simulink library "CTADP_lib"  (Simulink 7.5)
settings: Solver=ode45  StartTime=0.0  StopTime=10.0  RelTol=1e-3
libraries: simulink x2
settings Model: Creator=Yuri  LastModifiedBy=Yuri

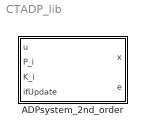
== system CTADP_lib ==
  ADPsystem_2nd_order : Subsystem  mask{K=[0,0], Q=eye(2), R=1, dT=0.1}
      mask prompts: K "Control gain K"; Q "Weight Matrix Q"; R "Weight Matrix R"; dT "Learning Interval dT"

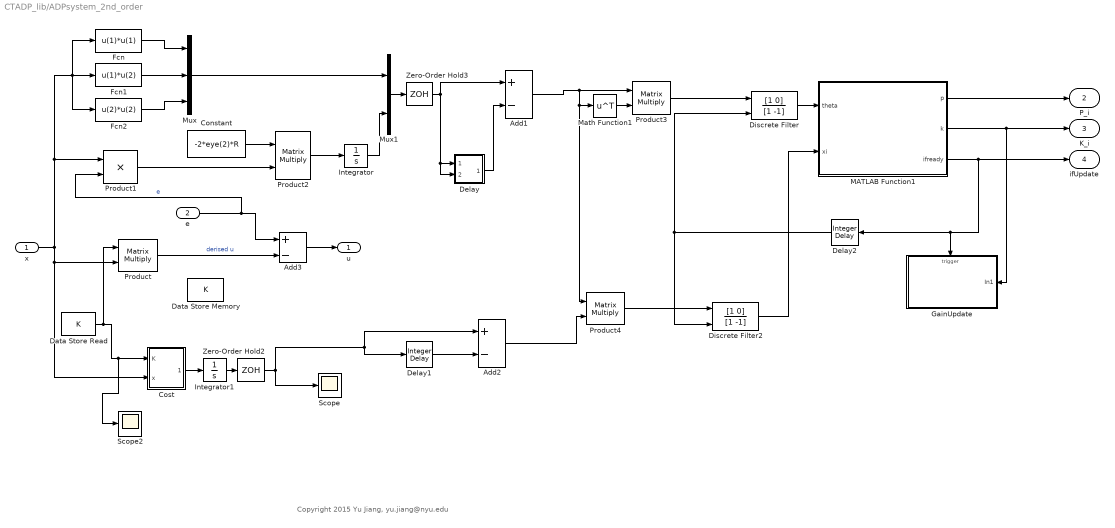
== system CTADP_lib/ADPsystem_2nd_order ==
  note: Copyright 2015 Yu Jiang, yu.jiang@nyu.edu
  x : Inport
  e : Inport  Port=2
  Add1 : Sum  Inputs=+-
  Add2 : Sum  Inputs=+-
  Add3 : Sum  Inputs=+-
  Constant : Constant  Value=-2*eye(2)*R  VectorParams1D=off
  Cost : Subsystem
  Data Store Memory : DataStoreMemory  Priority=1  DataStoreName=K  InitialValue=K  VectorParams1D=off
  Data Store Read : DataStoreRead  DataStoreName=K  SampleTime=0
  Delay : Subsystem  Description=Replaced Block
      mask Type: Replaced Block
      mask Description: SaveAs has replaced this block with an empty subsystem because the block represents a new type or uses a new functionality.
      mask Display: fprintf('Replaced: %s\n','Delay')
  Delay1 : simulink/Discrete/Integer Delay  NumDelays=1  vinit=0  samptime=dT
  Delay2 : simulink/Discrete/Integer Delay  NumDelays=1  vinit=0  samptime=dT
  Discrete Filter : DiscreteFilter  Numerator=[1 0]  Denominator=[1 -1]  SampleTime=dT  NumAccumDataTypeStr=Inherit: Same as product output  OutDataTypeStr=Inherit: Same as input
  Discrete Filter2 : DiscreteFilter  Numerator=[1 0]  Denominator=[1 -1]  SampleTime=dT  NumAccumDataTypeStr=Inherit: Same as product output  OutDataTypeStr=Inherit: Same as input
  Fcn : Fcn  Expr=u(1)*u(1)
  Fcn1 : Fcn  Expr=u(1)*u(2)
  Fcn2 : Fcn  Expr=u(2)*u(2)
  GainUpdate : Subsystem
  Integrator : Integrator
  Integrator1 : Integrator
  MATLAB Function1 : Stateflow chart  TreatAsAtomicUnit=on
      settings: PermitHierarchicalResolution=ParametersOnly
  Math Function1 : Math  Operator=transpose  SaturateOnIntegerOverflow=on
  Mux : Mux  Inputs=3
  Mux1 : Mux  Inputs=2
  Product{,2..4} (4 alike) : Product  Multiplication=Matrix(*)
  Product1 : Product
  Scope : Scope
  Scope2 : Scope
      settings: SaveName=ScopeData4
  Zero-Order Hold2 : ZeroOrderHold  SampleTime=dT
  Zero-Order Hold3 : ZeroOrderHold  SampleTime=dT
  u : Outport
  P_i : Outport  Port=2
  K_i : Outport  Port=3
  ifUpdate : Outport  Port=4
  wires:
  x/1 -> Cost/2(x), Product/2, Fcn/1, Fcn2/1, Fcn1/1, Product1/1
  Product/1 -> Add3/2  "derised u"
  Data Store Read/1 -> Scope2/1, Cost/1(K), Product/1
  Fcn1/1 -> Mux/2
  Fcn/1 -> Mux/1
  Fcn2/1 -> Mux/3
  Product1/1 -> Product2/2
  Constant/1 -> Product2/1
  Product2/1 -> Integrator/1
  Integrator/1 -> Mux1/2
  Zero-Order Hold3/1 -> Delay/2(In2), Delay/1(In1), Add1/1
  Mux/1 -> Mux1/1
  Delay/1(Out1) -> Add1/2
  Cost/1(r(x,uk)) -> Integrator1/1
  Integrator1/1 -> Zero-Order Hold2/1
  Delay1/1 -> Add2/2
  Add3/1 -> u/1
  e/1 -> Product1/2, Add3/1  "e"
  Math Function1/1 -> Product3/2
  Product3/1 -> Discrete Filter/1
  Add2/1 -> Product4/2
  Product4/1 -> Discrete Filter2/1
  Discrete Filter/1 -> MATLAB Function1/1(theta)
  Discrete Filter2/1 -> MATLAB Function1/2(xi)
  Mux1/1 -> Zero-Order Hold3/1
  Zero-Order Hold2/1 -> Scope/1, Delay1/1, Add2/1
  MATLAB Function1/3(ifready) -> ifUpdate/1, Delay2/1, GainUpdate/Trigger
  MATLAB Function1/1(p) -> P_i/1
  MATLAB Function1/2(k) -> GainUpdate/1(In1), K_i/1
  Delay2/1 -> Discrete Filter/2, Discrete Filter2/2
  Add1/1 -> Product4/1, Math Function1/1, Product3/1

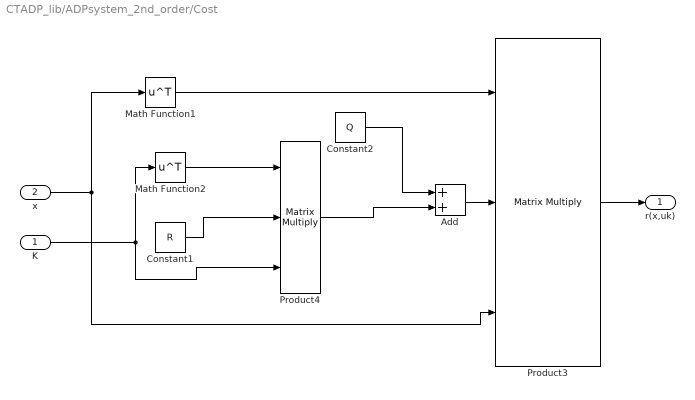
== system CTADP_lib/ADPsystem_2nd_order/Cost ==
  K : Inport
  x : Inport  Port=2
  Add : Sum
  Constant1 : Constant  Value=R
  Constant2 : Constant  Value=Q
  Math Function1 : Math  Operator=transpose  SaturateOnIntegerOverflow=on
  Math Function2 : Math  Operator=transpose  SaturateOnIntegerOverflow=on
  Product3 : Product  Inputs=3  Multiplication=Matrix(*)
  Product4 : Product  Inputs=3  Multiplication=Matrix(*)
  r(x,uk) : Outport
  wires:
  Add/1 -> Product3/2
  x/1 -> Math Function1/1, Product3/3
  Product4/1 -> Add/2
  Math Function1/1 -> Product3/1
  Product3/1 -> r(x,uk)/1
  Constant2/1 -> Add/1
  K/1 -> Math Function2/1, Product4/3
  Constant1/1 -> Product4/2
  Math Function2/1 -> Product4/1

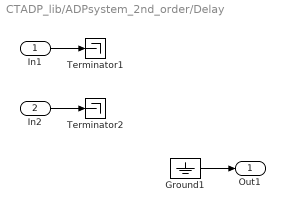
== system CTADP_lib/ADPsystem_2nd_order/Delay ==
  In1 : Inport
  In2 : Inport  Port=2
  Ground1 : Ground
  Terminator1 : Terminator
  Terminator2 : Terminator
  Out1 : Outport
  wires:
  Ground1/1 -> Out1/1
  In2/1 -> Terminator2/1
  In1/1 -> Terminator1/1

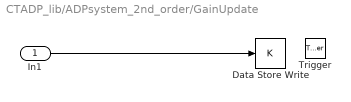
== system CTADP_lib/ADPsystem_2nd_order/GainUpdate ==
  In1 : Inport
  Trigger : TriggerPort  PortDimensions=1
  Data Store Write : DataStoreWrite  DataStoreName=K
  wires:
  In1/1 -> Data Store Write/1

== matlab function ADPsystem_2nd_order/MATLAB Function1 ==
  data: theta input double; p output double; k output double; xi input double; ifready output double
function [p,k,ifready] = fcn(theta,xi)
%#eml
ifready = (rank(theta)==5);

if ifready
 pv = -theta\xi;    
else
 pv = zeros(5,1);
end

 p = [pv(1) pv(2)/2; pv(2)/2 pv(3)];
 k = pv(4:5)';
end
